simulink model "dspUDPVoip"  (Simulink 8.3)
settings: Solver=FixedStepDiscrete  StartTime=0.0  StopTime=inf  RelTol=1e-3
libraries: dspsrcs4 x2, dspnetwork x2, dspmisc x1, dspsnks4 x1
settings Model: Creator=The MathWorks Inc.
settings OptimizationCC: ExpressionDepthLimit=2147483647
settings DebuggingCC: SolverPrmCheckMsg=none  FcnCallInpInsideContextMsg=UseLocalSettings  StrictBusMsg=Warning

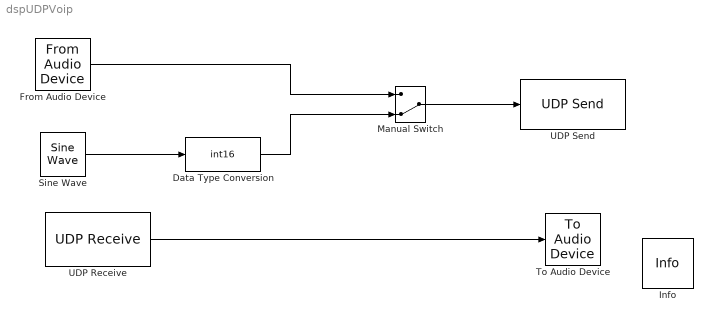
== system dspUDPVoip ==
  Data Type Conversion : DataTypeConversion  OutDataTypeStr=int16
  From Audio Device : dspsrcs4/From Audio Device  deviceName=Default  numChannels=1  sampleRate=44100  deviceDatatype=16-bit integer  autoBufferSize=on  bufferSize=4096  queueDuration=1.0  frameSize=1024  outputDatatype=int16  defaultInputChannelMapping=on  inputChannelMapping=1
  Info : dspmisc/Info  SystemSampleTime=-1
  Manual Switch : ManualSwitch  CurrentSetting=0
  Sine Wave : dspsrcs4/Sine Wave  Amplitude=2^15  Frequency=110  Phase=0  SampleMode=Discrete  OutComplex=Real  CompMethod=Trigonometric fcn  TableSize=Speed  SampleTime=1/44100  SamplesPerFrame=1024  ResetState=Restart at time zero  dataType=double  wordLen=16  udDataType=sfix(16)  fracBitsMode=Best precision  numFracBits=15  OutDataTypeStr=double  LastOutDataTypeStr=double
  To Audio Device : dspsnks4/To Audio Device  deviceName=Default  inheritSampleRate=on  sampleRate=44100  deviceDatatype=16-bit integer  autoBufferSize=on  bufferSize=4096  queueDuration=1.0  defaultOutputChannelMapping=on  outputChannelMapping=1
  UDP Receive : dspnetwork/UDP Receive  localURL='0.0.0.0'  localPort=5001  remoteURL='0.0.0.0'  remotePort=-1  recvBufferSize=8192  dims=1024  signalDatatype=int16  isVarSize=on  showBlockingTime=off  blockingTime=0  sampletime=1024/44100
  UDP Send : dspnetwork/UDP Send  remoteURL='127.0.0.1'  remotePort=5000  localURL='127.0.0.1'  localPortSource=Automatically determine  localPort=-1  sampletime=-1  separateLengthPort=0
  wires:
  From Audio Device/1 -> Manual Switch/1
  Sine Wave/1 -> Data Type Conversion/1
  Manual Switch/1 -> UDP Send/1
  Data Type Conversion/1 -> Manual Switch/2
  UDP Receive/1 -> To Audio Device/1
